simulink library "batteryModelFromCellSemiDetailed2RC"  (R2023a)
settings: Solver=VariableStepAuto  StartTime=0.0  StopTime=10.0  RelTol=1e-3
undefined symbols (not defined in the file or in its folder): battery_builder_rtmsupport, gcbh
libraries: batteryModelFromCellSemiDetailed2RC_lib x42
(part 1 of 2)
settings Model: Creator=paofu  LastModifiedBy=paofu

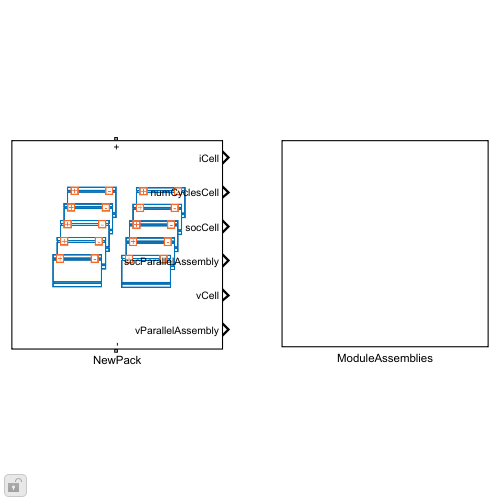
[thumbnail: Simulink's stored preview of the top-level diagram]
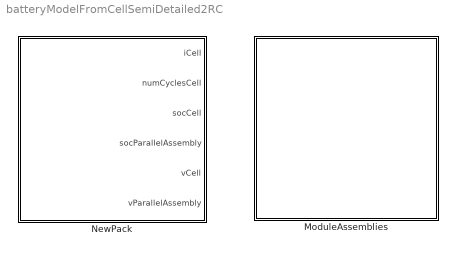
== system batteryModelFromCellSemiDetailed2RC ==
  ModuleAssemblies : Subsystem
  NewPack : Subsystem  LoadFcn=battery_builder_rtmsupport('loadfcn',gcbh);
      settings: CopyFcn=battery_builder_rtmsupport('copyfcn',gcbh);  PreCopyFcn=battery_builder_rtmsupport('precopyfcn',gcbh);  PreDeleteFcn=battery_builder_rtmsupport('predeletefcn',gcbh);  PortSchema="{\"entries\":[{\"content\":{\"sides\":[{\"content\":{\"connectorIds\":[\"LConn1\"]},\"type\":\"ConnectorPlacement.EquallySpacedRectSide\",\"uuid\":\"c12930f2-be9e-4fd5-b7ef-2c0d097eff71\"},{\"content\":{\"connectorIds\":[\"RConn1\"],\"side\":\"RIGHT\"},\"type\":\"ConnectorPlacement.EquallySpacedRectSide\",\"uuid\":\"9600c4b3-3abd-4358-9f10-7cc7281dc828\"},{\"content\":{\"side\":\"TOP\"},\"type\":\"ConnectorPlacement.EquallySpacedRectSide\",\"uuid\":\"039aee12-8f13-42ff-82bb-3b8cf5a1d5c9\"},{\"content\":{\"connectorIds\":[\"Out1\",\"Out2\",\"Out3\",\"Out4\",\"Out5\",\"Out6\"],\"side\":\"BOTTOM\"},\"type\":\"ConnectorPlacement.EquallySpacedRectSide\",\"uuid\":\"2cd3946a-0f37-4ab2-a76c-2a868876edc8\"}]},\"type\":\"ConnectorPlacement.EquallySpacedConnector\",\"uuid\":\"2e61461b-9c9d-464f-baa3-5ce2adcb4020\"}],\"packageUris\":[\"http://schema.mathworks.com/mf0/Connector/R2020b\"],\"version\":\"1.0\"}"
      mask Display: image('$imagefile')

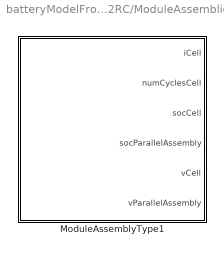
== system batteryModelFromCellSemiDetailed2RC/ModuleAssemblies ==
  ModuleAssemblyType1 : Subsystem  LoadFcn=battery_builder_rtmsupport('loadfcn',gcbh);
      settings: CopyFcn=battery_builder_rtmsupport('copyfcn',gcbh);  PreCopyFcn=battery_builder_rtmsupport('precopyfcn',gcbh);  PreDeleteFcn=battery_builder_rtmsupport('predeletefcn',gcbh);  PortSchema="{\"entries\":[{\"content\":{\"sides\":[{\"content\":{\"connectorIds\":[\"LConn1\"]},\"type\":\"ConnectorPlacement.EquallySpacedRectSide\",\"uuid\":\"c12930f2-be9e-4fd5-b7ef-2c0d097eff71\"},{\"content\":{\"connectorIds\":[\"RConn1\"],\"side\":\"RIGHT\"},\"type\":\"ConnectorPlacement.EquallySpacedRectSide\",\"uuid\":\"9600c4b3-3abd-4358-9f10-7cc7281dc828\"},{\"content\":{\"side\":\"TOP\"},\"type\":\"ConnectorPlacement.EquallySpacedRectSide\",\"uuid\":\"039aee12-8f13-42ff-82bb-3b8cf5a1d5c9\"},{\"content\":{\"connectorIds\":[\"Out1\",\"Out2\",\"Out3\",\"Out4\",\"Out5\",\"Out6\"],\"side\":\"BOTTOM\"},\"type\":\"ConnectorPlacement.EquallySpacedRectSide\",\"uuid\":\"b469a464-f429-4be9-9e4d-c22d413aa1f4\"}]},\"type\":\"ConnectorPlacement.EquallySpacedConnector\",\"uuid\":\"2e61461b-9c9d-464f-baa3-5ce2adcb4020\"}],\"packageUris\":[\"http://schema.mathworks.com/mf0/Connector/R2020b\"],\"version\":\"1.0\"}"
      mask Display: image('$imagefile')

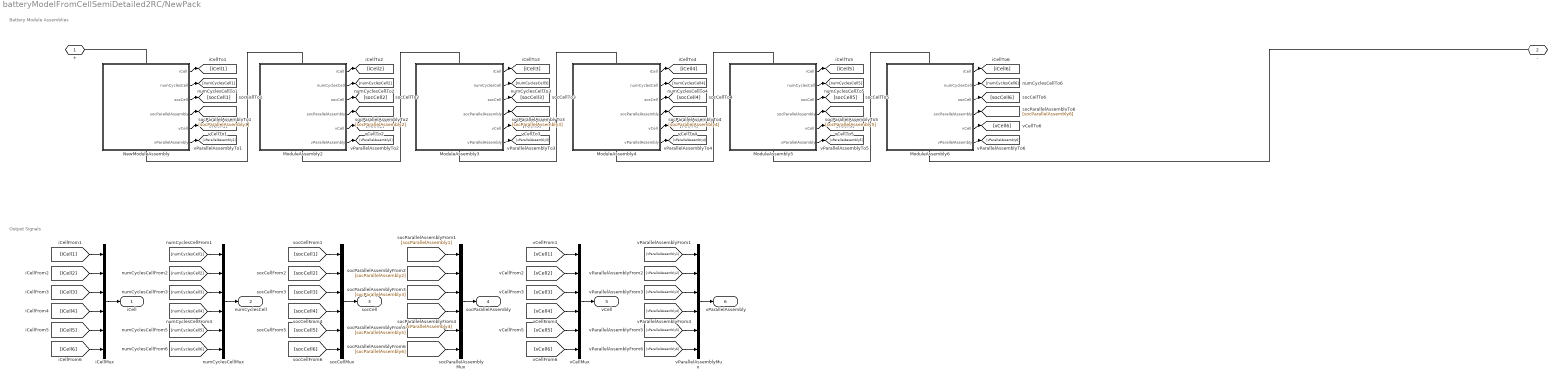
== system batteryModelFromCellSemiDetailed2RC/NewPack ==
  note: Battery Module Assemblies
  note: Output Signals
  ModuleAssembly2 : Subsystem  LoadFcn=battery_builder_rtmsupport('loadfcn',gcbh);
      settings: CopyFcn=battery_builder_rtmsupport('copyfcn',gcbh);  PreCopyFcn=battery_builder_rtmsupport('precopyfcn',gcbh);  PreDeleteFcn=battery_builder_rtmsupport('predeletefcn',gcbh);  PortSchema="{\"entries\":[{\"content\":{\"sides\":[{\"content\":{\"connectorIds\":[\"LConn1\"]},\"type\":\"ConnectorPlacement.EquallySpacedRectSide\",\"uuid\":\"c12930f2-be9e-4fd5-b7ef-2c0d097eff71\"},{\"content\":{\"connectorIds\":[\"RConn1\"],\"side\":\"RIGHT\"},\"type\":\"ConnectorPlacement.EquallySpacedRectSide\",\"uuid\":\"9600c4b3-3abd-4358-9f10-7cc7281dc828\"},{\"content\":{\"side\":\"TOP\"},\"type\":\"ConnectorPlacement.EquallySpacedRectSide\",\"uuid\":\"039aee12-8f13-42ff-82bb-3b8cf5a1d5c9\"},{\"content\":{\"connectorIds\":[\"Out1\",\"Out2\",\"Out3\",\"Out4\",\"Out5\",\"Out6\"],\"side\":\"BOTTOM\"},\"type\":\"ConnectorPlacement.EquallySpacedRectSide\",\"uuid\":\"b469a464-f429-4be9-9e4d-c22d413aa1f4\"}]},\"type\":\"ConnectorPlacement.EquallySpacedConnector\",\"uuid\":\"2e61461b-9c9d-464f-baa3-5ce2adcb4020\"}],\"packageUris\":[\"http://schema.mathworks.com/mf0/Connector/R2020b\"],\"version\":\"1.0\"}"
      mask Display: image('$imagefile')
  ModuleAssembly3 : Subsystem  LoadFcn=battery_builder_rtmsupport('loadfcn',gcbh);
      settings: CopyFcn=battery_builder_rtmsupport('copyfcn',gcbh);  PreCopyFcn=battery_builder_rtmsupport('precopyfcn',gcbh);  PreDeleteFcn=battery_builder_rtmsupport('predeletefcn',gcbh);  PortSchema="{\"entries\":[{\"content\":{\"sides\":[{\"content\":{\"connectorIds\":[\"LConn1\"]},\"type\":\"ConnectorPlacement.EquallySpacedRectSide\",\"uuid\":\"c12930f2-be9e-4fd5-b7ef-2c0d097eff71\"},{\"content\":{\"connectorIds\":[\"RConn1\"],\"side\":\"RIGHT\"},\"type\":\"ConnectorPlacement.EquallySpacedRectSide\",\"uuid\":\"9600c4b3-3abd-4358-9f10-7cc7281dc828\"},{\"content\":{\"side\":\"TOP\"},\"type\":\"ConnectorPlacement.EquallySpacedRectSide\",\"uuid\":\"039aee12-8f13-42ff-82bb-3b8cf5a1d5c9\"},{\"content\":{\"connectorIds\":[\"Out1\",\"Out2\",\"Out3\",\"Out4\",\"Out5\",\"Out6\"],\"side\":\"BOTTOM\"},\"type\":\"ConnectorPlacement.EquallySpacedRectSide\",\"uuid\":\"b469a464-f429-4be9-9e4d-c22d413aa1f4\"}]},\"type\":\"ConnectorPlacement.EquallySpacedConnector\",\"uuid\":\"2e61461b-9c9d-464f-baa3-5ce2adcb4020\"}],\"packageUris\":[\"http://schema.mathworks.com/mf0/Connector/R2020b\"],\"version\":\"1.0\"}"
      mask Display: image('$imagefile')
  ModuleAssembly4 : Subsystem  LoadFcn=battery_builder_rtmsupport('loadfcn',gcbh);
      settings: CopyFcn=battery_builder_rtmsupport('copyfcn',gcbh);  PreCopyFcn=battery_builder_rtmsupport('precopyfcn',gcbh);  PreDeleteFcn=battery_builder_rtmsupport('predeletefcn',gcbh);  PortSchema="{\"entries\":[{\"content\":{\"sides\":[{\"content\":{\"connectorIds\":[\"LConn1\"]},\"type\":\"ConnectorPlacement.EquallySpacedRectSide\",\"uuid\":\"c12930f2-be9e-4fd5-b7ef-2c0d097eff71\"},{\"content\":{\"connectorIds\":[\"RConn1\"],\"side\":\"RIGHT\"},\"type\":\"ConnectorPlacement.EquallySpacedRectSide\",\"uuid\":\"9600c4b3-3abd-4358-9f10-7cc7281dc828\"},{\"content\":{\"side\":\"TOP\"},\"type\":\"ConnectorPlacement.EquallySpacedRectSide\",\"uuid\":\"039aee12-8f13-42ff-82bb-3b8cf5a1d5c9\"},{\"content\":{\"connectorIds\":[\"Out1\",\"Out2\",\"Out3\",\"Out4\",\"Out5\",\"Out6\"],\"side\":\"BOTTOM\"},\"type\":\"ConnectorPlacement.EquallySpacedRectSide\",\"uuid\":\"b469a464-f429-4be9-9e4d-c22d413aa1f4\"}]},\"type\":\"ConnectorPlacement.EquallySpacedConnector\",\"uuid\":\"2e61461b-9c9d-464f-baa3-5ce2adcb4020\"}],\"packageUris\":[\"http://schema.mathworks.com/mf0/Connector/R2020b\"],\"version\":\"1.0\"}"
      mask Display: image('$imagefile')
  ModuleAssembly5 : Subsystem  LoadFcn=battery_builder_rtmsupport('loadfcn',gcbh);
      settings: CopyFcn=battery_builder_rtmsupport('copyfcn',gcbh);  PreCopyFcn=battery_builder_rtmsupport('precopyfcn',gcbh);  PreDeleteFcn=battery_builder_rtmsupport('predeletefcn',gcbh);  PortSchema="{\"entries\":[{\"content\":{\"sides\":[{\"content\":{\"connectorIds\":[\"LConn1\"]},\"type\":\"ConnectorPlacement.EquallySpacedRectSide\",\"uuid\":\"c12930f2-be9e-4fd5-b7ef-2c0d097eff71\"},{\"content\":{\"connectorIds\":[\"RConn1\"],\"side\":\"RIGHT\"},\"type\":\"ConnectorPlacement.EquallySpacedRectSide\",\"uuid\":\"9600c4b3-3abd-4358-9f10-7cc7281dc828\"},{\"content\":{\"side\":\"TOP\"},\"type\":\"ConnectorPlacement.EquallySpacedRectSide\",\"uuid\":\"039aee12-8f13-42ff-82bb-3b8cf5a1d5c9\"},{\"content\":{\"connectorIds\":[\"Out1\",\"Out2\",\"Out3\",\"Out4\",\"Out5\",\"Out6\"],\"side\":\"BOTTOM\"},\"type\":\"ConnectorPlacement.EquallySpacedRectSide\",\"uuid\":\"b469a464-f429-4be9-9e4d-c22d413aa1f4\"}]},\"type\":\"ConnectorPlacement.EquallySpacedConnector\",\"uuid\":\"2e61461b-9c9d-464f-baa3-5ce2adcb4020\"}],\"packageUris\":[\"http://schema.mathworks.com/mf0/Connector/R2020b\"],\"version\":\"1.0\"}"
      mask Display: image('$imagefile')
  ModuleAssembly6 : Subsystem  LoadFcn=battery_builder_rtmsupport('loadfcn',gcbh);
      settings: CopyFcn=battery_builder_rtmsupport('copyfcn',gcbh);  PreCopyFcn=battery_builder_rtmsupport('precopyfcn',gcbh);  PreDeleteFcn=battery_builder_rtmsupport('predeletefcn',gcbh);  PortSchema="{\"entries\":[{\"content\":{\"sides\":[{\"content\":{\"connectorIds\":[\"LConn1\"]},\"type\":\"ConnectorPlacement.EquallySpacedRectSide\",\"uuid\":\"c12930f2-be9e-4fd5-b7ef-2c0d097eff71\"},{\"content\":{\"connectorIds\":[\"RConn1\"],\"side\":\"RIGHT\"},\"type\":\"ConnectorPlacement.EquallySpacedRectSide\",\"uuid\":\"9600c4b3-3abd-4358-9f10-7cc7281dc828\"},{\"content\":{\"side\":\"TOP\"},\"type\":\"ConnectorPlacement.EquallySpacedRectSide\",\"uuid\":\"039aee12-8f13-42ff-82bb-3b8cf5a1d5c9\"},{\"content\":{\"connectorIds\":[\"Out1\",\"Out2\",\"Out3\",\"Out4\",\"Out5\",\"Out6\"],\"side\":\"BOTTOM\"},\"type\":\"ConnectorPlacement.EquallySpacedRectSide\",\"uuid\":\"b469a464-f429-4be9-9e4d-c22d413aa1f4\"}]},\"type\":\"ConnectorPlacement.EquallySpacedConnector\",\"uuid\":\"2e61461b-9c9d-464f-baa3-5ce2adcb4020\"}],\"packageUris\":[\"http://schema.mathworks.com/mf0/Connector/R2020b\"],\"version\":\"1.0\"}"
      mask Display: image('$imagefile')
  NewModuleAssembly : Subsystem  LoadFcn=battery_builder_rtmsupport('loadfcn',gcbh);
      settings: CopyFcn=battery_builder_rtmsupport('copyfcn',gcbh);  PreCopyFcn=battery_builder_rtmsupport('precopyfcn',gcbh);  PreDeleteFcn=battery_builder_rtmsupport('predeletefcn',gcbh);  PortSchema="{\"entries\":[{\"content\":{\"sides\":[{\"content\":{\"connectorIds\":[\"LConn1\"]},\"type\":\"ConnectorPlacement.EquallySpacedRectSide\",\"uuid\":\"c12930f2-be9e-4fd5-b7ef-2c0d097eff71\"},{\"content\":{\"connectorIds\":[\"RConn1\"],\"side\":\"RIGHT\"},\"type\":\"ConnectorPlacement.EquallySpacedRectSide\",\"uuid\":\"9600c4b3-3abd-4358-9f10-7cc7281dc828\"},{\"content\":{\"side\":\"TOP\"},\"type\":\"ConnectorPlacement.EquallySpacedRectSide\",\"uuid\":\"039aee12-8f13-42ff-82bb-3b8cf5a1d5c9\"},{\"content\":{\"connectorIds\":[\"Out1\",\"Out2\",\"Out3\",\"Out4\",\"Out5\",\"Out6\"],\"side\":\"BOTTOM\"},\"type\":\"ConnectorPlacement.EquallySpacedRectSide\",\"uuid\":\"b469a464-f429-4be9-9e4d-c22d413aa1f4\"}]},\"type\":\"ConnectorPlacement.EquallySpacedConnector\",\"uuid\":\"2e61461b-9c9d-464f-baa3-5ce2adcb4020\"}],\"packageUris\":[\"http://schema.mathworks.com/mf0/Connector/R2020b\"],\"version\":\"1.0\"}"
      mask Display: image('$imagefile')
  iCellMux : Mux  Inputs=6
  numCyclesCellMux : Mux  Inputs=6
  socCellMux : Mux  Inputs=6
  socParallelAssemblyMux : Mux  Inputs=6
  vCellMux : Mux  Inputs=6
  vParallelAssemblyMux : Mux  Inputs=6
  + : PMIOPort  Side=Left
  - : PMIOPort  Port=2  Side=Right
  iCell : Outport
  numCyclesCell : Outport  Port=2
  socCell : Outport  Port=3
  socParallelAssembly : Outport  Port=4
  vCell : Outport  Port=5
  vParallelAssembly : Outport  Port=6
  wires:
  NewModuleAssembly/1(iCell) -> [iCell1]
  iCellMux/1 -> iCell/1
  [iCell1] -> iCellMux/1
  NewModuleAssembly/2(numCyclesCell) -> [numCyclesCell1]
  numCyclesCellMux/1 -> numCyclesCell/1
  [numCyclesCell1] -> numCyclesCellMux/1
  NewModuleAssembly/3(socCell) -> [socCell1]
  socCellMux/1 -> socCell/1
  [socCell1] -> socCellMux/1
  NewModuleAssembly/4(socParallelAssembly) -> [socParallelAssembly1]
  socParallelAssemblyMux/1 -> socParallelAssembly/1
  [socParallelAssembly1] -> socParallelAssemblyMux/1
  NewModuleAssembly/5(vCell) -> [vCell1]
  vCellMux/1 -> vCell/1
  [vCell1] -> vCellMux/1
  NewModuleAssembly/6(vParallelAssembly) -> [vParallelAssembly1]
  vParallelAssemblyMux/1 -> vParallelAssembly/1
  [vParallelAssembly1] -> vParallelAssemblyMux/1
  ModuleAssembly2/1(iCell) -> [iCell2]
  [iCell2] -> iCellMux/2
  ModuleAssembly2/2(numCyclesCell) -> [numCyclesCell2]
  [numCyclesCell2] -> numCyclesCellMux/2
  ModuleAssembly2/3(socCell) -> [socCell2]
  [socCell2] -> socCellMux/2
  ModuleAssembly2/4(socParallelAssembly) -> [socParallelAssembly2]
  [socParallelAssembly2] -> socParallelAssemblyMux/2
  ModuleAssembly2/5(vCell) -> [vCell2]
  [vCell2] -> vCellMux/2
  ModuleAssembly2/6(vParallelAssembly) -> [vParallelAssembly2]
  [vParallelAssembly2] -> vParallelAssemblyMux/2
  ModuleAssembly3/1(iCell) -> [iCell3]
  [iCell3] -> iCellMux/3
  ModuleAssembly3/2(numCyclesCell) -> [numCyclesCell3]
  [numCyclesCell3] -> numCyclesCellMux/3
  ModuleAssembly3/3(socCell) -> [socCell3]
  [socCell3] -> socCellMux/3
  ModuleAssembly3/4(socParallelAssembly) -> [socParallelAssembly3]
  [socParallelAssembly3] -> socParallelAssemblyMux/3
  ModuleAssembly3/5(vCell) -> [vCell3]
  [vCell3] -> vCellMux/3
  ModuleAssembly3/6(vParallelAssembly) -> [vParallelAssembly3]
  [vParallelAssembly3] -> vParallelAssemblyMux/3
  ModuleAssembly4/1(iCell) -> [iCell4]
  [iCell4] -> iCellMux/4
  ModuleAssembly4/2(numCyclesCell) -> [numCyclesCell4]
  [numCyclesCell4] -> numCyclesCellMux/4
  ModuleAssembly4/3(socCell) -> [socCell4]
  [socCell4] -> socCellMux/4
  ModuleAssembly4/4(socParallelAssembly) -> [socParallelAssembly4]
  [socParallelAssembly4] -> socParallelAssemblyMux/4
  ModuleAssembly4/5(vCell) -> [vCell4]
  [vCell4] -> vCellMux/4
  ModuleAssembly4/6(vParallelAssembly) -> [vParallelAssembly4]
  [vParallelAssembly4] -> vParallelAssemblyMux/4
  ModuleAssembly5/1(iCell) -> [iCell5]
  [iCell5] -> iCellMux/5
  ModuleAssembly5/2(numCyclesCell) -> [numCyclesCell5]
  [numCyclesCell5] -> numCyclesCellMux/5
  ModuleAssembly5/3(socCell) -> [socCell5]
  [socCell5] -> socCellMux/5
  ModuleAssembly5/4(socParallelAssembly) -> [socParallelAssembly5]
  [socParallelAssembly5] -> socParallelAssemblyMux/5
  ModuleAssembly5/5(vCell) -> [vCell5]
  [vCell5] -> vCellMux/5
  ModuleAssembly5/6(vParallelAssembly) -> [vParallelAssembly5]
  [vParallelAssembly5] -> vParallelAssemblyMux/5
  ModuleAssembly6/1(iCell) -> [iCell6]
  [iCell6] -> iCellMux/6
  ModuleAssembly6/2(numCyclesCell) -> [numCyclesCell6]
  [numCyclesCell6] -> numCyclesCellMux/6
  ModuleAssembly6/3(socCell) -> [socCell6]
  [socCell6] -> socCellMux/6
  ModuleAssembly6/4(socParallelAssembly) -> [socParallelAssembly6]
  [socParallelAssembly6] -> socParallelAssemblyMux/6
  ModuleAssembly6/5(vCell) -> [vCell6]
  [vCell6] -> vCellMux/6
  ModuleAssembly6/6(vParallelAssembly) -> [vParallelAssembly6]
  [vParallelAssembly6] -> vParallelAssemblyMux/6
  connections:
  ModuleAssembly2/LConn1 -- NewModuleAssembly/RConn1
  ModuleAssembly3/LConn1 -- ModuleAssembly2/RConn1
  ModuleAssembly4/LConn1 -- ModuleAssembly3/RConn1
  ModuleAssembly5/LConn1 -- ModuleAssembly4/RConn1
  ModuleAssembly6/LConn1 -- ModuleAssembly5/RConn1
  NewModuleAssembly/LConn1 -- +/RConn1
  ModuleAssembly6/RConn1 -- -/RConn1

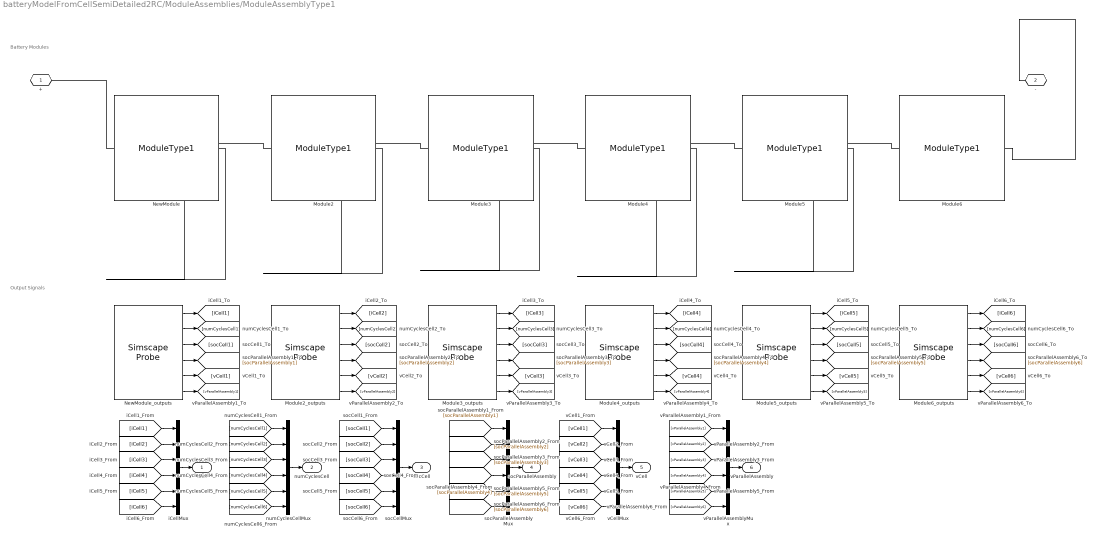
== system batteryModelFromCellSemiDetailed2RC/ModuleAssemblies/ModuleAssemblyType1 ==
  note: Battery Modules
  note: Output Signals
  Module{2..6} (5 alike) : batteryModelFromCellSemiDetailed2RC_lib/Modules/ModuleType1  SOC_vecCell=ModuleType1.SOC_vecCell  V0_vecCell=ModuleType1.V0_vecCell V  V_rangeCell=ModuleType1.V_rangeCell V  R0_vecCell=ModuleType1.R0_vecCell Ohm  AHCell=ModuleType1.AHCell A*hr  extrapolation_optionCell=simscape.enum.extrapolation.nearest  R1_vecCell=ModuleType1.R1_vecCell Ohm  tau1_vecCell=ModuleType1.tau1_vecCell s  R2_vecCell=ModuleType1.R2_vecCell Ohm  tau2_vecCell=ModuleType1.tau2_vecCell s  P=4  S=3  iCell_specify=off  iCell_priority=None  iCell=0 A  iCell_nominal_specify=off  iCell_nominal_unit=A  iCell_nominal_value=1  vCell_specify=off  vCell_priority=None  vCell=0 V  vCell_nominal_specify=off  vCell_nominal_unit=V  vCell_nominal_value=1  socCell_specify=off  socCell_priority=High  socCell=1  socCell_nominal_specify=off  socCell_nominal_unit=1  socCell_nominal_value=1  numCyclesCell_specify=off  numCyclesCell_priority=High  numCyclesCell=0  numCyclesCell_nominal_specify=off  numCyclesCell_nominal_unit=1  numCyclesCell_nominal_value=1  vParallelAssembly_specify=off  vParallelAssembly_priority=None  vParallelAssembly=repmat(0, 3, 1) V  vParallelAssembly_nominal_specify=off  vParallelAssembly_nominal_unit=V  vParallelAssembly_nominal_value=1  socParallelAssembly_specify=off  socParallelAssembly_priority=None  socParallelAssembly=repmat(1, 3, 1)  socParallelAssembly_nominal_specify=off  socParallelAssembly_nominal_unit=1  socParallelAssembly_nominal_value=1
      settings: InternalSimscapePortConfiguration="{\"Bottom\":[{\"id\":\"n\",\"label\":\"-\",\"type\":\"foundation.electrical.electrical\"}],\"Left\":[],\"Right\":[],\"Top\":[{\"id\":\"p\",\"label\":\"+\",\"type\":\"foundation.electrical.electrical\"}]}"
  Module2_outputs : SimscapeProbe  BoundBlock=4  Variables={iCell, numCyclesCell, socCell, socParallelAssembly, vCell, vParallelAssembly}
  Module3_outputs : SimscapeProbe  BoundBlock=5  Variables={iCell, numCyclesCell, socCell, socParallelAssembly, vCell, vParallelAssembly}
  Module4_outputs : SimscapeProbe  BoundBlock=6  Variables={iCell, numCyclesCell, socCell, socParallelAssembly, vCell, vParallelAssembly}
  Module5_outputs : SimscapeProbe  BoundBlock=7  Variables={iCell, numCyclesCell, socCell, socParallelAssembly, vCell, vParallelAssembly}
  Module6_outputs : SimscapeProbe  BoundBlock=8  Variables={iCell, numCyclesCell, socCell, socParallelAssembly, vCell, vParallelAssembly}
  NewModule : batteryModelFromCellSemiDetailed2RC_lib/Modules/ModuleType1  SOC_vecCell=ModuleType1.SOC_vecCell  V0_vecCell=ModuleType1.V0_vecCell V  V_rangeCell=ModuleType1.V_rangeCell V  R0_vecCell=ModuleType1.R0_vecCell Ohm  AHCell=ModuleType1.AHCell A*hr  extrapolation_optionCell=simscape.enum.extrapolation.nearest  R1_vecCell=ModuleType1.R1_vecCell Ohm  tau1_vecCell=ModuleType1.tau1_vecCell s  R2_vecCell=ModuleType1.R2_vecCell Ohm  tau2_vecCell=ModuleType1.tau2_vecCell s  P=4  S=3  iCell_specify=off  iCell_priority=None  iCell=0 A  iCell_nominal_specify=off  iCell_nominal_unit=A  iCell_nominal_value=1  vCell_specify=off  vCell_priority=None  vCell=0 V  vCell_nominal_specify=off  vCell_nominal_unit=V  vCell_nominal_value=1  socCell_specify=off  socCell_priority=High  socCell=1  socCell_nominal_specify=off  socCell_nominal_unit=1  socCell_nominal_value=1  numCyclesCell_specify=off  numCyclesCell_priority=High  numCyclesCell=0  numCyclesCell_nominal_specify=off  numCyclesCell_nominal_unit=1  numCyclesCell_nominal_value=1  vParallelAssembly_specify=off  vParallelAssembly_priority=None  vParallelAssembly=repmat(0, 3, 1) V  vParallelAssembly_nominal_specify=off  vParallelAssembly_nominal_unit=V  vParallelAssembly_nominal_value=1  socParallelAssembly_specify=off  socParallelAssembly_priority=None  socParallelAssembly=repmat(1, 3, 1)  socParallelAssembly_nominal_specify=off  socParallelAssembly_nominal_unit=1  socParallelAssembly_nominal_value=1
      settings: InternalSimscapePortConfiguration="{\"Bottom\":[{\"id\":\"n\",\"label\":\"-\",\"type\":\"foundation.electrical.electrical\"}],\"Left\":[],\"Right\":[],\"Top\":[{\"id\":\"p\",\"label\":\"+\",\"type\":\"foundation.electrical.electrical\"}]}"
  NewModule_outputs : SimscapeProbe  BoundBlock=3  Variables={iCell, numCyclesCell, socCell, socParallelAssembly, vCell, vParallelAssembly}
  iCellMux : Mux  Inputs=6
  numCyclesCellMux : Mux  Inputs=6
  socCellMux : Mux  Inputs=6
  socParallelAssemblyMux : Mux  Inputs=6
  vCellMux : Mux  Inputs=6
  vParallelAssemblyMux : Mux  Inputs=6
  + : PMIOPort  Side=Left
  - : PMIOPort  Port=2  Side=Right
  iCell : Outport
  numCyclesCell : Outport  Port=2
  socCell : Outport  Port=3
  socParallelAssembly : Outport  Port=4
  vCell : Outport  Port=5
  vParallelAssembly : Outport  Port=6
  wires:
  NewModule_outputs/1 -> [iCell1]
  iCellMux/1 -> iCell/1
  [iCell1] -> iCellMux/1
  NewModule_outputs/2 -> [numCyclesCell1]
  numCyclesCellMux/1 -> numCyclesCell/1
  [numCyclesCell1] -> numCyclesCellMux/1
  NewModule_outputs/3 -> [socCell1]
  socCellMux/1 -> socCell/1
  [socCell1] -> socCellMux/1
  NewModule_outputs/4 -> [socParallelAssembly1]
  socParallelAssemblyMux/1 -> socParallelAssembly/1
  [socParallelAssembly1] -> socParallelAssemblyMux/1
  NewModule_outputs/5 -> [vCell1]
  vCellMux/1 -> vCell/1
  [vCell1] -> vCellMux/1
  NewModule_outputs/6 -> [vParallelAssembly1]
  vParallelAssemblyMux/1 -> vParallelAssembly/1
  [vParallelAssembly1] -> vParallelAssemblyMux/1
  Module2_outputs/1 -> [iCell2]
  [iCell2] -> iCellMux/2
  Module2_outputs/2 -> [numCyclesCell2]
  [numCyclesCell2] -> numCyclesCellMux/2
  Module2_outputs/3 -> [socCell2]
  [socCell2] -> socCellMux/2
  Module2_outputs/4 -> [socParallelAssembly2]
  [socParallelAssembly2] -> socParallelAssemblyMux/2
  Module2_outputs/5 -> [vCell2]
  [vCell2] -> vCellMux/2
  Module2_outputs/6 -> [vParallelAssembly2]
  [vParallelAssembly2] -> vParallelAssemblyMux/2
  Module3_outputs/1 -> [iCell3]
  [iCell3] -> iCellMux/3
  Module3_outputs/2 -> [numCyclesCell3]
  [numCyclesCell3] -> numCyclesCellMux/3
  Module3_outputs/3 -> [socCell3]
  [socCell3] -> socCellMux/3
  Module3_outputs/4 -> [socParallelAssembly3]
  [socParallelAssembly3] -> socParallelAssemblyMux/3
  Module3_outputs/5 -> [vCell3]
  [vCell3] -> vCellMux/3
  Module3_outputs/6 -> [vParallelAssembly3]
  [vParallelAssembly3] -> vParallelAssemblyMux/3
  Module4_outputs/1 -> [iCell4]
  [iCell4] -> iCellMux/4
  Module4_outputs/2 -> [numCyclesCell4]
  [numCyclesCell4] -> numCyclesCellMux/4
  Module4_outputs/3 -> [socCell4]
  [socCell4] -> socCellMux/4
  Module4_outputs/4 -> [socParallelAssembly4]
  [socParallelAssembly4] -> socParallelAssemblyMux/4
  Module4_outputs/5 -> [vCell4]
  [vCell4] -> vCellMux/4
  Module4_outputs/6 -> [vParallelAssembly4]
  [vParallelAssembly4] -> vParallelAssemblyMux/4
  Module5_outputs/1 -> [iCell5]
  [iCell5] -> iCellMux/5
  Module5_outputs/2 -> [numCyclesCell5]
  [numCyclesCell5] -> numCyclesCellMux/5
  Module5_outputs/3 -> [socCell5]
  [socCell5] -> socCellMux/5
  Module5_outputs/4 -> [socParallelAssembly5]
  [socParallelAssembly5] -> socParallelAssemblyMux/5
  Module5_outputs/5 -> [vCell5]
  [vCell5] -> vCellMux/5
  Module5_outputs/6 -> [vParallelAssembly5]
  [vParallelAssembly5] -> vParallelAssemblyMux/5
  Module6_outputs/1 -> [iCell6]
  [iCell6] -> iCellMux/6
  Module6_outputs/2 -> [numCyclesCell6]
  [numCyclesCell6] -> numCyclesCellMux/6
  Module6_outputs/3 -> [socCell6]
  [socCell6] -> socCellMux/6
  Module6_outputs/4 -> [socParallelAssembly6]
  [socParallelAssembly6] -> socParallelAssemblyMux/6
  Module6_outputs/5 -> [vCell6]
  [vCell6] -> vCellMux/6
  Module6_outputs/6 -> [vParallelAssembly6]
  [vParallelAssembly6] -> vParallelAssemblyMux/6
  connections:
  Module2/LConn1 -- NewModule/RConn1
  Module3/LConn1 -- Module2/RConn1
  Module4/LConn1 -- Module3/RConn1
  Module5/LConn1 -- Module4/RConn1
  Module6/LConn1 -- Module5/RConn1
  NewModule/LConn1 -- +/RConn1
  Module6/RConn1 -- -/RConn1

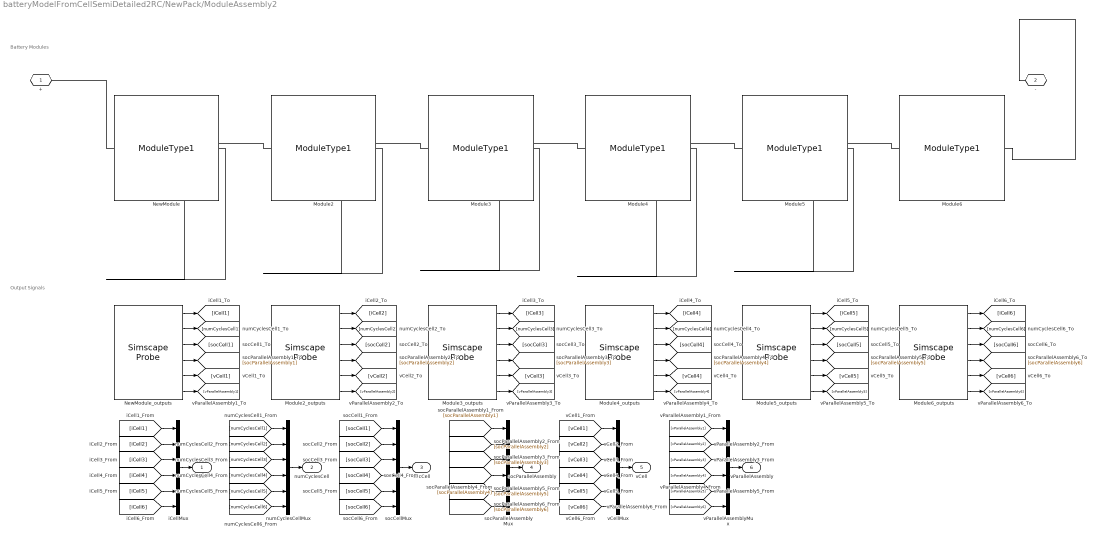
== system batteryModelFromCellSemiDetailed2RC/NewPack/ModuleAssembly2 ==
  note: Output Signals
  note: Battery Modules
  Module{2..6} (5 alike) : batteryModelFromCellSemiDetailed2RC_lib/Modules/ModuleType1  SOC_vecCell=ModuleType1.SOC_vecCell  V0_vecCell=ModuleType1.V0_vecCell V  V_rangeCell=ModuleType1.V_rangeCell V  R0_vecCell=ModuleType1.R0_vecCell Ohm  AHCell=ModuleType1.AHCell A*hr  extrapolation_optionCell=simscape.enum.extrapolation.nearest  R1_vecCell=ModuleType1.R1_vecCell Ohm  tau1_vecCell=ModuleType1.tau1_vecCell s  R2_vecCell=ModuleType1.R2_vecCell Ohm  tau2_vecCell=ModuleType1.tau2_vecCell s  P=4  S=3  iCell_specify=off  iCell_priority=None  iCell=0 A  iCell_nominal_specify=off  iCell_nominal_unit=A  iCell_nominal_value=1  vCell_specify=off  vCell_priority=None  vCell=0 V  vCell_nominal_specify=off  vCell_nominal_unit=V  vCell_nominal_value=1  socCell_specify=off  socCell_priority=High  socCell=1  socCell_nominal_specify=off  socCell_nominal_unit=1  socCell_nominal_value=1  numCyclesCell_specify=off  numCyclesCell_priority=High  numCyclesCell=0  numCyclesCell_nominal_specify=off  numCyclesCell_nominal_unit=1  numCyclesCell_nominal_value=1  vParallelAssembly_specify=off  vParallelAssembly_priority=None  vParallelAssembly=repmat(0, 3, 1) V  vParallelAssembly_nominal_specify=off  vParallelAssembly_nominal_unit=V  vParallelAssembly_nominal_value=1  socParallelAssembly_specify=off  socParallelAssembly_priority=None  socParallelAssembly=repmat(1, 3, 1)  socParallelAssembly_nominal_specify=off  socParallelAssembly_nominal_unit=1  socParallelAssembly_nominal_value=1
      settings: InternalSimscapePortConfiguration="{\"Bottom\":[{\"id\":\"n\",\"label\":\"-\",\"type\":\"foundation.electrical.electrical\"}],\"Left\":[],\"Right\":[],\"Top\":[{\"id\":\"p\",\"label\":\"+\",\"type\":\"foundation.electrical.electrical\"}]}"
  Module2_outputs : SimscapeProbe  BoundBlock=206  Variables={iCell, numCyclesCell, socCell, socParallelAssembly, vCell, vParallelAssembly}
  Module3_outputs : SimscapeProbe  BoundBlock=208  Variables={iCell, numCyclesCell, socCell, socParallelAssembly, vCell, vParallelAssembly}
  Module4_outputs : SimscapeProbe  BoundBlock=210  Variables={iCell, numCyclesCell, socCell, socParallelAssembly, vCell, vParallelAssembly}
  Module5_outputs : SimscapeProbe  BoundBlock=212  Variables={iCell, numCyclesCell, socCell, socParallelAssembly, vCell, vParallelAssembly}
  Module6_outputs : SimscapeProbe  BoundBlock=214  Variables={iCell, numCyclesCell, socCell, socParallelAssembly, vCell, vParallelAssembly}
  NewModule : batteryModelFromCellSemiDetailed2RC_lib/Modules/ModuleType1  SOC_vecCell=ModuleType1.SOC_vecCell  V0_vecCell=ModuleType1.V0_vecCell V  V_rangeCell=ModuleType1.V_rangeCell V  R0_vecCell=ModuleType1.R0_vecCell Ohm  AHCell=ModuleType1.AHCell A*hr  extrapolation_optionCell=simscape.enum.extrapolation.nearest  R1_vecCell=ModuleType1.R1_vecCell Ohm  tau1_vecCell=ModuleType1.tau1_vecCell s  R2_vecCell=ModuleType1.R2_vecCell Ohm  tau2_vecCell=ModuleType1.tau2_vecCell s  P=4  S=3  iCell_specify=off  iCell_priority=None  iCell=0 A  iCell_nominal_specify=off  iCell_nominal_unit=A  iCell_nominal_value=1  vCell_specify=off  vCell_priority=None  vCell=0 V  vCell_nominal_specify=off  vCell_nominal_unit=V  vCell_nominal_value=1  socCell_specify=off  socCell_priority=High  socCell=1  socCell_nominal_specify=off  socCell_nominal_unit=1  socCell_nominal_value=1  numCyclesCell_specify=off  numCyclesCell_priority=High  numCyclesCell=0  numCyclesCell_nominal_specify=off  numCyclesCell_nominal_unit=1  numCyclesCell_nominal_value=1  vParallelAssembly_specify=off  vParallelAssembly_priority=None  vParallelAssembly=repmat(0, 3, 1) V  vParallelAssembly_nominal_specify=off  vParallelAssembly_nominal_unit=V  vParallelAssembly_nominal_value=1  socParallelAssembly_specify=off  socParallelAssembly_priority=None  socParallelAssembly=repmat(1, 3, 1)  socParallelAssembly_nominal_specify=off  socParallelAssembly_nominal_unit=1  socParallelAssembly_nominal_value=1
      settings: InternalSimscapePortConfiguration="{\"Bottom\":[{\"id\":\"n\",\"label\":\"-\",\"type\":\"foundation.electrical.electrical\"}],\"Left\":[],\"Right\":[],\"Top\":[{\"id\":\"p\",\"label\":\"+\",\"type\":\"foundation.electrical.electrical\"}]}"
  NewModule_outputs : SimscapeProbe  BoundBlock=216  Variables={iCell, numCyclesCell, socCell, socParallelAssembly, vCell, vParallelAssembly}
  iCellMux : Mux  Inputs=6
  numCyclesCellMux : Mux  Inputs=6
  socCellMux : Mux  Inputs=6
  socParallelAssemblyMux : Mux  Inputs=6
  vCellMux : Mux  Inputs=6
  vParallelAssemblyMux : Mux  Inputs=6
  + : PMIOPort  Side=Left
  - : PMIOPort  Port=2  Side=Right
  iCell : Outport
  numCyclesCell : Outport  Port=2
  socCell : Outport  Port=3
  socParallelAssembly : Outport  Port=4
  vCell : Outport  Port=5
  vParallelAssembly : Outport  Port=6
  wires:
  [vParallelAssembly6] -> vParallelAssemblyMux/6
  Module6_outputs/6 -> [vParallelAssembly6]
  [vCell6] -> vCellMux/6
  Module6_outputs/5 -> [vCell6]
  [socParallelAssembly6] -> socParallelAssemblyMux/6
  Module6_outputs/4 -> [socParallelAssembly6]
  [socCell6] -> socCellMux/6
  Module6_outputs/3 -> [socCell6]
  [numCyclesCell6] -> numCyclesCellMux/6
  Module6_outputs/2 -> [numCyclesCell6]
  [iCell6] -> iCellMux/6
  Module6_outputs/1 -> [iCell6]
  [vParallelAssembly5] -> vParallelAssemblyMux/5
  Module5_outputs/6 -> [vParallelAssembly5]
  [vCell5] -> vCellMux/5
  Module5_outputs/5 -> [vCell5]
  [socParallelAssembly5] -> socParallelAssemblyMux/5
  Module5_outputs/4 -> [socParallelAssembly5]
  [socCell5] -> socCellMux/5
  Module5_outputs/3 -> [socCell5]
  [numCyclesCell5] -> numCyclesCellMux/5
  Module5_outputs/2 -> [numCyclesCell5]
  [iCell5] -> iCellMux/5
  Module5_outputs/1 -> [iCell5]
  [vParallelAssembly4] -> vParallelAssemblyMux/4
  Module4_outputs/6 -> [vParallelAssembly4]
  [vCell4] -> vCellMux/4
  Module4_outputs/5 -> [vCell4]
  [socParallelAssembly4] -> socParallelAssemblyMux/4
  Module4_outputs/4 -> [socParallelAssembly4]
  [socCell4] -> socCellMux/4
  Module4_outputs/3 -> [socCell4]
  [numCyclesCell4] -> numCyclesCellMux/4
  Module4_outputs/2 -> [numCyclesCell4]
  [iCell4] -> iCellMux/4
  Module4_outputs/1 -> [iCell4]
  [vParallelAssembly3] -> vParallelAssemblyMux/3
  Module3_outputs/6 -> [vParallelAssembly3]
  [vCell3] -> vCellMux/3
  Module3_outputs/5 -> [vCell3]
  [socParallelAssembly3] -> socParallelAssemblyMux/3
  Module3_outputs/4 -> [socParallelAssembly3]
  [socCell3] -> socCellMux/3
  Module3_outputs/3 -> [socCell3]
  [numCyclesCell3] -> numCyclesCellMux/3
  Module3_outputs/2 -> [numCyclesCell3]
  [iCell3] -> iCellMux/3
  Module3_outputs/1 -> [iCell3]
  [vParallelAssembly2] -> vParallelAssemblyMux/2
  Module2_outputs/6 -> [vParallelAssembly2]
  [vCell2] -> vCellMux/2
  Module2_outputs/5 -> [vCell2]
  [socParallelAssembly2] -> socParallelAssemblyMux/2
  Module2_outputs/4 -> [socParallelAssembly2]
  [socCell2] -> socCellMux/2
  Module2_outputs/3 -> [socCell2]
  [numCyclesCell2] -> numCyclesCellMux/2
  Module2_outputs/2 -> [numCyclesCell2]
  [iCell2] -> iCellMux/2
  Module2_outputs/1 -> [iCell2]
  [vParallelAssembly1] -> vParallelAssemblyMux/1
  vParallelAssemblyMux/1 -> vParallelAssembly/1
  NewModule_outputs/6 -> [vParallelAssembly1]
  [vCell1] -> vCellMux/1
  vCellMux/1 -> vCell/1
  NewModule_outputs/5 -> [vCell1]
  [socParallelAssembly1] -> socParallelAssemblyMux/1
  socParallelAssemblyMux/1 -> socParallelAssembly/1
  NewModule_outputs/4 -> [socParallelAssembly1]
  [socCell1] -> socCellMux/1
  socCellMux/1 -> socCell/1
  NewModule_outputs/3 -> [socCell1]
  [numCyclesCell1] -> numCyclesCellMux/1
  numCyclesCellMux/1 -> numCyclesCell/1
  NewModule_outputs/2 -> [numCyclesCell1]
  [iCell1] -> iCellMux/1
  iCellMux/1 -> iCell/1
  NewModule_outputs/1 -> [iCell1]
  connections:
  Module6/RConn1 -- -/RConn1
  NewModule/LConn1 -- +/RConn1
  Module6/LConn1 -- Module5/RConn1
  Module5/LConn1 -- Module4/RConn1
  Module4/LConn1 -- Module3/RConn1
  Module3/LConn1 -- Module2/RConn1
  Module2/LConn1 -- NewModule/RConn1

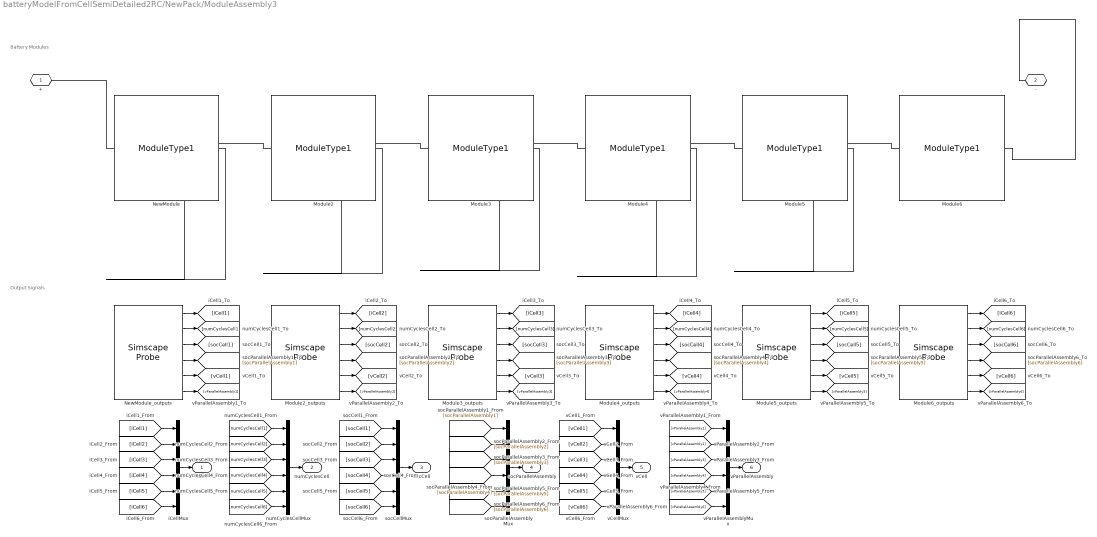
== system batteryModelFromCellSemiDetailed2RC/NewPack/ModuleAssembly3 ==
  note: Output Signals
  note: Battery Modules
  Module{2..6} (5 alike) : batteryModelFromCellSemiDetailed2RC_lib/Modules/ModuleType1  SOC_vecCell=ModuleType1.SOC_vecCell  V0_vecCell=ModuleType1.V0_vecCell V  V_rangeCell=ModuleType1.V_rangeCell V  R0_vecCell=ModuleType1.R0_vecCell Ohm  AHCell=ModuleType1.AHCell A*hr  extrapolation_optionCell=simscape.enum.extrapolation.nearest  R1_vecCell=ModuleType1.R1_vecCell Ohm  tau1_vecCell=ModuleType1.tau1_vecCell s  R2_vecCell=ModuleType1.R2_vecCell Ohm  tau2_vecCell=ModuleType1.tau2_vecCell s  P=4  S=3  iCell_specify=off  iCell_priority=None  iCell=0 A  iCell_nominal_specify=off  iCell_nominal_unit=A  iCell_nominal_value=1  vCell_specify=off  vCell_priority=None  vCell=0 V  vCell_nominal_specify=off  vCell_nominal_unit=V  vCell_nominal_value=1  socCell_specify=off  socCell_priority=High  socCell=1  socCell_nominal_specify=off  socCell_nominal_unit=1  socCell_nominal_value=1  numCyclesCell_specify=off  numCyclesCell_priority=High  numCyclesCell=0  numCyclesCell_nominal_specify=off  numCyclesCell_nominal_unit=1  numCyclesCell_nominal_value=1  vParallelAssembly_specify=off  vParallelAssembly_priority=None  vParallelAssembly=repmat(0, 3, 1) V  vParallelAssembly_nominal_specify=off  vParallelAssembly_nominal_unit=V  vParallelAssembly_nominal_value=1  socParallelAssembly_specify=off  socParallelAssembly_priority=None  socParallelAssembly=repmat(1, 3, 1)  socParallelAssembly_nominal_specify=off  socParallelAssembly_nominal_unit=1  socParallelAssembly_nominal_value=1
      settings: InternalSimscapePortConfiguration="{\"Bottom\":[{\"id\":\"n\",\"label\":\"-\",\"type\":\"foundation.electrical.electrical\"}],\"Left\":[],\"Right\":[],\"Top\":[{\"id\":\"p\",\"label\":\"+\",\"type\":\"foundation.electrical.electrical\"}]}"
  Module2_outputs : SimscapeProbe  BoundBlock=307  Variables={iCell, numCyclesCell, socCell, socParallelAssembly, vCell, vParallelAssembly}
  Module3_outputs : SimscapeProbe  BoundBlock=309  Variables={iCell, numCyclesCell, socCell, socParallelAssembly, vCell, vParallelAssembly}
  Module4_outputs : SimscapeProbe  BoundBlock=311  Variables={iCell, numCyclesCell, socCell, socParallelAssembly, vCell, vParallelAssembly}
  Module5_outputs : SimscapeProbe  BoundBlock=313  Variables={iCell, numCyclesCell, socCell, socParallelAssembly, vCell, vParallelAssembly}
  Module6_outputs : SimscapeProbe  BoundBlock=315  Variables={iCell, numCyclesCell, socCell, socParallelAssembly, vCell, vParallelAssembly}
  NewModule : batteryModelFromCellSemiDetailed2RC_lib/Modules/ModuleType1  SOC_vecCell=ModuleType1.SOC_vecCell  V0_vecCell=ModuleType1.V0_vecCell V  V_rangeCell=ModuleType1.V_rangeCell V  R0_vecCell=ModuleType1.R0_vecCell Ohm  AHCell=ModuleType1.AHCell A*hr  extrapolation_optionCell=simscape.enum.extrapolation.nearest  R1_vecCell=ModuleType1.R1_vecCell Ohm  tau1_vecCell=ModuleType1.tau1_vecCell s  R2_vecCell=ModuleType1.R2_vecCell Ohm  tau2_vecCell=ModuleType1.tau2_vecCell s  P=4  S=3  iCell_specify=off  iCell_priority=None  iCell=0 A  iCell_nominal_specify=off  iCell_nominal_unit=A  iCell_nominal_value=1  vCell_specify=off  vCell_priority=None  vCell=0 V  vCell_nominal_specify=off  vCell_nominal_unit=V  vCell_nominal_value=1  socCell_specify=off  socCell_priority=High  socCell=1  socCell_nominal_specify=off  socCell_nominal_unit=1  socCell_nominal_value=1  numCyclesCell_specify=off  numCyclesCell_priority=High  numCyclesCell=0  numCyclesCell_nominal_specify=off  numCyclesCell_nominal_unit=1  numCyclesCell_nominal_value=1  vParallelAssembly_specify=off  vParallelAssembly_priority=None  vParallelAssembly=repmat(0, 3, 1) V  vParallelAssembly_nominal_specify=off  vParallelAssembly_nominal_unit=V  vParallelAssembly_nominal_value=1  socParallelAssembly_specify=off  socParallelAssembly_priority=None  socParallelAssembly=repmat(1, 3, 1)  socParallelAssembly_nominal_specify=off  socParallelAssembly_nominal_unit=1  socParallelAssembly_nominal_value=1
      settings: InternalSimscapePortConfiguration="{\"Bottom\":[{\"id\":\"n\",\"label\":\"-\",\"type\":\"foundation.electrical.electrical\"}],\"Left\":[],\"Right\":[],\"Top\":[{\"id\":\"p\",\"label\":\"+\",\"type\":\"foundation.electrical.electrical\"}]}"
  NewModule_outputs : SimscapeProbe  BoundBlock=317  Variables={iCell, numCyclesCell, socCell, socParallelAssembly, vCell, vParallelAssembly}
  iCellMux : Mux  Inputs=6
  numCyclesCellMux : Mux  Inputs=6
  socCellMux : Mux  Inputs=6
  socParallelAssemblyMux : Mux  Inputs=6
  vCellMux : Mux  Inputs=6
  vParallelAssemblyMux : Mux  Inputs=6
  + : PMIOPort  Side=Left
  - : PMIOPort  Port=2  Side=Right
  iCell : Outport
  numCyclesCell : Outport  Port=2
  socCell : Outport  Port=3
  socParallelAssembly : Outport  Port=4
  vCell : Outport  Port=5
  vParallelAssembly : Outport  Port=6
  wires:
  [vParallelAssembly6] -> vParallelAssemblyMux/6
  Module6_outputs/6 -> [vParallelAssembly6]
  [vCell6] -> vCellMux/6
  Module6_outputs/5 -> [vCell6]
  [socParallelAssembly6] -> socParallelAssemblyMux/6
  Module6_outputs/4 -> [socParallelAssembly6]
  [socCell6] -> socCellMux/6
  Module6_outputs/3 -> [socCell6]
  [numCyclesCell6] -> numCyclesCellMux/6
  Module6_outputs/2 -> [numCyclesCell6]
  [iCell6] -> iCellMux/6
  Module6_outputs/1 -> [iCell6]
  [vParallelAssembly5] -> vParallelAssemblyMux/5
  Module5_outputs/6 -> [vParallelAssembly5]
  [vCell5] -> vCellMux/5
  Module5_outputs/5 -> [vCell5]
  [socParallelAssembly5] -> socParallelAssemblyMux/5
  Module5_outputs/4 -> [socParallelAssembly5]
  [socCell5] -> socCellMux/5
  Module5_outputs/3 -> [socCell5]
  [numCyclesCell5] -> numCyclesCellMux/5
  Module5_outputs/2 -> [numCyclesCell5]
  [iCell5] -> iCellMux/5
  Module5_outputs/1 -> [iCell5]
  [vParallelAssembly4] -> vParallelAssemblyMux/4
  Module4_outputs/6 -> [vParallelAssembly4]
  [vCell4] -> vCellMux/4
  Module4_outputs/5 -> [vCell4]
  [socParallelAssembly4] -> socParallelAssemblyMux/4
  Module4_outputs/4 -> [socParallelAssembly4]
  [socCell4] -> socCellMux/4
  Module4_outputs/3 -> [socCell4]
  [numCyclesCell4] -> numCyclesCellMux/4
  Module4_outputs/2 -> [numCyclesCell4]
  [iCell4] -> iCellMux/4
  Module4_outputs/1 -> [iCell4]
  [vParallelAssembly3] -> vParallelAssemblyMux/3
  Module3_outputs/6 -> [vParallelAssembly3]
  [vCell3] -> vCellMux/3
  Module3_outputs/5 -> [vCell3]
  [socParallelAssembly3] -> socParallelAssemblyMux/3
  Module3_outputs/4 -> [socParallelAssembly3]
  [socCell3] -> socCellMux/3
  Module3_outputs/3 -> [socCell3]
  [numCyclesCell3] -> numCyclesCellMux/3
  Module3_outputs/2 -> [numCyclesCell3]
  [iCell3] -> iCellMux/3
  Module3_outputs/1 -> [iCell3]
  [vParallelAssembly2] -> vParallelAssemblyMux/2
  Module2_outputs/6 -> [vParallelAssembly2]
  [vCell2] -> vCellMux/2
  Module2_outputs/5 -> [vCell2]
  [socParallelAssembly2] -> socParallelAssemblyMux/2
  Module2_outputs/4 -> [socParallelAssembly2]
  [socCell2] -> socCellMux/2
  Module2_outputs/3 -> [socCell2]
  [numCyclesCell2] -> numCyclesCellMux/2
  Module2_outputs/2 -> [numCyclesCell2]
  [iCell2] -> iCellMux/2
  Module2_outputs/1 -> [iCell2]
  [vParallelAssembly1] -> vParallelAssemblyMux/1
  vParallelAssemblyMux/1 -> vParallelAssembly/1
  NewModule_outputs/6 -> [vParallelAssembly1]
  [vCell1] -> vCellMux/1
  vCellMux/1 -> vCell/1
  NewModule_outputs/5 -> [vCell1]
  [socParallelAssembly1] -> socParallelAssemblyMux/1
  socParallelAssemblyMux/1 -> socParallelAssembly/1
  NewModule_outputs/4 -> [socParallelAssembly1]
  [socCell1] -> socCellMux/1
  socCellMux/1 -> socCell/1
  NewModule_outputs/3 -> [socCell1]
  [numCyclesCell1] -> numCyclesCellMux/1
  numCyclesCellMux/1 -> numCyclesCell/1
  NewModule_outputs/2 -> [numCyclesCell1]
  [iCell1] -> iCellMux/1
  iCellMux/1 -> iCell/1
  NewModule_outputs/1 -> [iCell1]
  connections:
  Module6/RConn1 -- -/RConn1
  NewModule/LConn1 -- +/RConn1
  Module6/LConn1 -- Module5/RConn1
  Module5/LConn1 -- Module4/RConn1
  Module4/LConn1 -- Module3/RConn1
  Module3/LConn1 -- Module2/RConn1
  Module2/LConn1 -- NewModule/RConn1

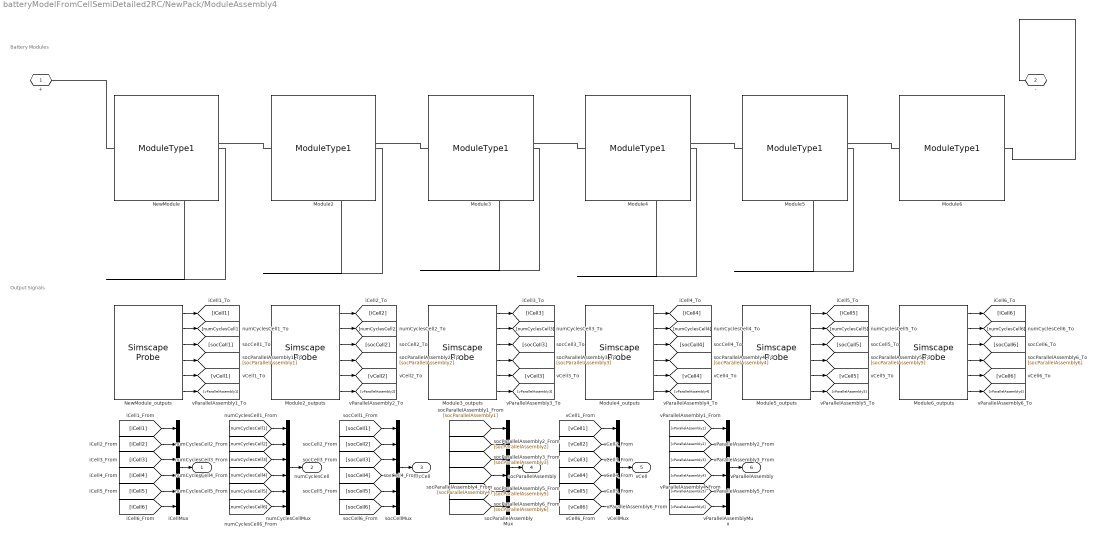
== system batteryModelFromCellSemiDetailed2RC/NewPack/ModuleAssembly4 ==
  note: Output Signals
  note: Battery Modules
  Module{2..6} (5 alike) : batteryModelFromCellSemiDetailed2RC_lib/Modules/ModuleType1  SOC_vecCell=ModuleType1.SOC_vecCell  V0_vecCell=ModuleType1.V0_vecCell V  V_rangeCell=ModuleType1.V_rangeCell V  R0_vecCell=ModuleType1.R0_vecCell Ohm  AHCell=ModuleType1.AHCell A*hr  extrapolation_optionCell=simscape.enum.extrapolation.nearest  R1_vecCell=ModuleType1.R1_vecCell Ohm  tau1_vecCell=ModuleType1.tau1_vecCell s  R2_vecCell=ModuleType1.R2_vecCell Ohm  tau2_vecCell=ModuleType1.tau2_vecCell s  P=4  S=3  iCell_specify=off  iCell_priority=None  iCell=0 A  iCell_nominal_specify=off  iCell_nominal_unit=A  iCell_nominal_value=1  vCell_specify=off  vCell_priority=None  vCell=0 V  vCell_nominal_specify=off  vCell_nominal_unit=V  vCell_nominal_value=1  socCell_specify=off  socCell_priority=High  socCell=1  socCell_nominal_specify=off  socCell_nominal_unit=1  socCell_nominal_value=1  numCyclesCell_specify=off  numCyclesCell_priority=High  numCyclesCell=0  numCyclesCell_nominal_specify=off  numCyclesCell_nominal_unit=1  numCyclesCell_nominal_value=1  vParallelAssembly_specify=off  vParallelAssembly_priority=None  vParallelAssembly=repmat(0, 3, 1) V  vParallelAssembly_nominal_specify=off  vParallelAssembly_nominal_unit=V  vParallelAssembly_nominal_value=1  socParallelAssembly_specify=off  socParallelAssembly_priority=None  socParallelAssembly=repmat(1, 3, 1)  socParallelAssembly_nominal_specify=off  socParallelAssembly_nominal_unit=1  socParallelAssembly_nominal_value=1
      settings: InternalSimscapePortConfiguration="{\"Bottom\":[{\"id\":\"n\",\"label\":\"-\",\"type\":\"foundation.electrical.electrical\"}],\"Left\":[],\"Right\":[],\"Top\":[{\"id\":\"p\",\"label\":\"+\",\"type\":\"foundation.electrical.electrical\"}]}"
  Module2_outputs : SimscapeProbe  BoundBlock=408  Variables={iCell, numCyclesCell, socCell, socParallelAssembly, vCell, vParallelAssembly}
  Module3_outputs : SimscapeProbe  BoundBlock=410  Variables={iCell, numCyclesCell, socCell, socParallelAssembly, vCell, vParallelAssembly}
  Module4_outputs : SimscapeProbe  BoundBlock=412  Variables={iCell, numCyclesCell, socCell, socParallelAssembly, vCell, vParallelAssembly}
  Module5_outputs : SimscapeProbe  BoundBlock=414  Variables={iCell, numCyclesCell, socCell, socParallelAssembly, vCell, vParallelAssembly}
  Module6_outputs : SimscapeProbe  BoundBlock=416  Variables={iCell, numCyclesCell, socCell, socParallelAssembly, vCell, vParallelAssembly}
  NewModule : batteryModelFromCellSemiDetailed2RC_lib/Modules/ModuleType1  SOC_vecCell=ModuleType1.SOC_vecCell  V0_vecCell=ModuleType1.V0_vecCell V  V_rangeCell=ModuleType1.V_rangeCell V  R0_vecCell=ModuleType1.R0_vecCell Ohm  AHCell=ModuleType1.AHCell A*hr  extrapolation_optionCell=simscape.enum.extrapolation.nearest  R1_vecCell=ModuleType1.R1_vecCell Ohm  tau1_vecCell=ModuleType1.tau1_vecCell s  R2_vecCell=ModuleType1.R2_vecCell Ohm  tau2_vecCell=ModuleType1.tau2_vecCell s  P=4  S=3  iCell_specify=off  iCell_priority=None  iCell=0 A  iCell_nominal_specify=off  iCell_nominal_unit=A  iCell_nominal_value=1  vCell_specify=off  vCell_priority=None  vCell=0 V  vCell_nominal_specify=off  vCell_nominal_unit=V  vCell_nominal_value=1  socCell_specify=off  socCell_priority=High  socCell=1  socCell_nominal_specify=off  socCell_nominal_unit=1  socCell_nominal_value=1  numCyclesCell_specify=off  numCyclesCell_priority=High  numCyclesCell=0  numCyclesCell_nominal_specify=off  numCyclesCell_nominal_unit=1  numCyclesCell_nominal_value=1  vParallelAssembly_specify=off  vParallelAssembly_priority=None  vParallelAssembly=repmat(0, 3, 1) V  vParallelAssembly_nominal_specify=off  vParallelAssembly_nominal_unit=V  vParallelAssembly_nominal_value=1  socParallelAssembly_specify=off  socParallelAssembly_priority=None  socParallelAssembly=repmat(1, 3, 1)  socParallelAssembly_nominal_specify=off  socParallelAssembly_nominal_unit=1  socParallelAssembly_nominal_value=1
      settings: InternalSimscapePortConfiguration="{\"Bottom\":[{\"id\":\"n\",\"label\":\"-\",\"type\":\"foundation.electrical.electrical\"}],\"Left\":[],\"Right\":[],\"Top\":[{\"id\":\"p\",\"label\":\"+\",\"type\":\"foundation.electrical.electrical\"}]}"
  NewModule_outputs : SimscapeProbe  BoundBlock=418  Variables={iCell, numCyclesCell, socCell, socParallelAssembly, vCell, vParallelAssembly}
  iCellMux : Mux  Inputs=6
  numCyclesCellMux : Mux  Inputs=6
  socCellMux : Mux  Inputs=6
  socParallelAssemblyMux : Mux  Inputs=6
  vCellMux : Mux  Inputs=6
  vParallelAssemblyMux : Mux  Inputs=6
  + : PMIOPort  Side=Left
  - : PMIOPort  Port=2  Side=Right
  iCell : Outport
  numCyclesCell : Outport  Port=2
  socCell : Outport  Port=3
  socParallelAssembly : Outport  Port=4
  vCell : Outport  Port=5
  vParallelAssembly : Outport  Port=6
  wires:
  [vParallelAssembly6] -> vParallelAssemblyMux/6
  Module6_outputs/6 -> [vParallelAssembly6]
  [vCell6] -> vCellMux/6
  Module6_outputs/5 -> [vCell6]
  [socParallelAssembly6] -> socParallelAssemblyMux/6
  Module6_outputs/4 -> [socParallelAssembly6]
  [socCell6] -> socCellMux/6
  Module6_outputs/3 -> [socCell6]
  [numCyclesCell6] -> numCyclesCellMux/6
  Module6_outputs/2 -> [numCyclesCell6]
  [iCell6] -> iCellMux/6
  Module6_outputs/1 -> [iCell6]
  [vParallelAssembly5] -> vParallelAssemblyMux/5
  Module5_outputs/6 -> [vParallelAssembly5]
  [vCell5] -> vCellMux/5
  Module5_outputs/5 -> [vCell5]
  [socParallelAssembly5] -> socParallelAssemblyMux/5
  Module5_outputs/4 -> [socParallelAssembly5]
  [socCell5] -> socCellMux/5
  Module5_outputs/3 -> [socCell5]
  [numCyclesCell5] -> numCyclesCellMux/5
  Module5_outputs/2 -> [numCyclesCell5]
  [iCell5] -> iCellMux/5
  Module5_outputs/1 -> [iCell5]
  [vParallelAssembly4] -> vParallelAssemblyMux/4
  Module4_outputs/6 -> [vParallelAssembly4]
  [vCell4] -> vCellMux/4
  Module4_outputs/5 -> [vCell4]
  [socParallelAssembly4] -> socParallelAssemblyMux/4
  Module4_outputs/4 -> [socParallelAssembly4]
  [socCell4] -> socCellMux/4
  Module4_outputs/3 -> [socCell4]
  [numCyclesCell4] -> numCyclesCellMux/4
  Module4_outputs/2 -> [numCyclesCell4]
  [iCell4] -> iCellMux/4
  Module4_outputs/1 -> [iCell4]
  [vParallelAssembly3] -> vParallelAssemblyMux/3
  Module3_outputs/6 -> [vParallelAssembly3]
  [vCell3] -> vCellMux/3
  Module3_outputs/5 -> [vCell3]
  [socParallelAssembly3] -> socParallelAssemblyMux/3
  Module3_outputs/4 -> [socParallelAssembly3]
  [socCell3] -> socCellMux/3
  Module3_outputs/3 -> [socCell3]
  [numCyclesCell3] -> numCyclesCellMux/3
  Module3_outputs/2 -> [numCyclesCell3]
  [iCell3] -> iCellMux/3
  Module3_outputs/1 -> [iCell3]
  [vParallelAssembly2] -> vParallelAssemblyMux/2
  Module2_outputs/6 -> [vParallelAssembly2]
  [vCell2] -> vCellMux/2
  Module2_outputs/5 -> [vCell2]
  [socParallelAssembly2] -> socParallelAssemblyMux/2
  Module2_outputs/4 -> [socParallelAssembly2]
  [socCell2] -> socCellMux/2
  Module2_outputs/3 -> [socCell2]
  [numCyclesCell2] -> numCyclesCellMux/2
  Module2_outputs/2 -> [numCyclesCell2]
  [iCell2] -> iCellMux/2
  Module2_outputs/1 -> [iCell2]
  [vParallelAssembly1] -> vParallelAssemblyMux/1
  vParallelAssemblyMux/1 -> vParallelAssembly/1
  NewModule_outputs/6 -> [vParallelAssembly1]
  [vCell1] -> vCellMux/1
  vCellMux/1 -> vCell/1
  NewModule_outputs/5 -> [vCell1]
  [socParallelAssembly1] -> socParallelAssemblyMux/1
  socParallelAssemblyMux/1 -> socParallelAssembly/1
  NewModule_outputs/4 -> [socParallelAssembly1]
  [socCell1] -> socCellMux/1
  socCellMux/1 -> socCell/1
  NewModule_outputs/3 -> [socCell1]
  [numCyclesCell1] -> numCyclesCellMux/1
  numCyclesCellMux/1 -> numCyclesCell/1
  NewModule_outputs/2 -> [numCyclesCell1]
  [iCell1] -> iCellMux/1
  iCellMux/1 -> iCell/1
  NewModule_outputs/1 -> [iCell1]
  connections:
  Module6/RConn1 -- -/RConn1
  NewModule/LConn1 -- +/RConn1
  Module6/LConn1 -- Module5/RConn1
  Module5/LConn1 -- Module4/RConn1
  Module4/LConn1 -- Module3/RConn1
  Module3/LConn1 -- Module2/RConn1
  Module2/LConn1 -- NewModule/RConn1
